simulink model "Twin_Rotor_Mimo_System_Pitch and Yaw Control"  (R2022b)
settings: Solver=VariableStepAuto  StartTime=0.0  StopTime=600
libraries: slpidlib x2
settings Model: SimulationMode=accelerator  Creator=Shaan Sapru  LastModifiedBy=Shaan Sapru
settings SolverCC: ZeroCrossAlgorithm=Adaptive
settings DebuggingCC: IgnoredZcDiagnostic=none

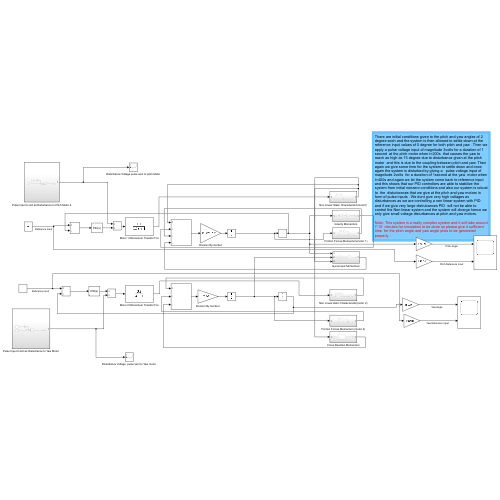
[thumbnail: Simulink's stored preview of the top-level diagram]
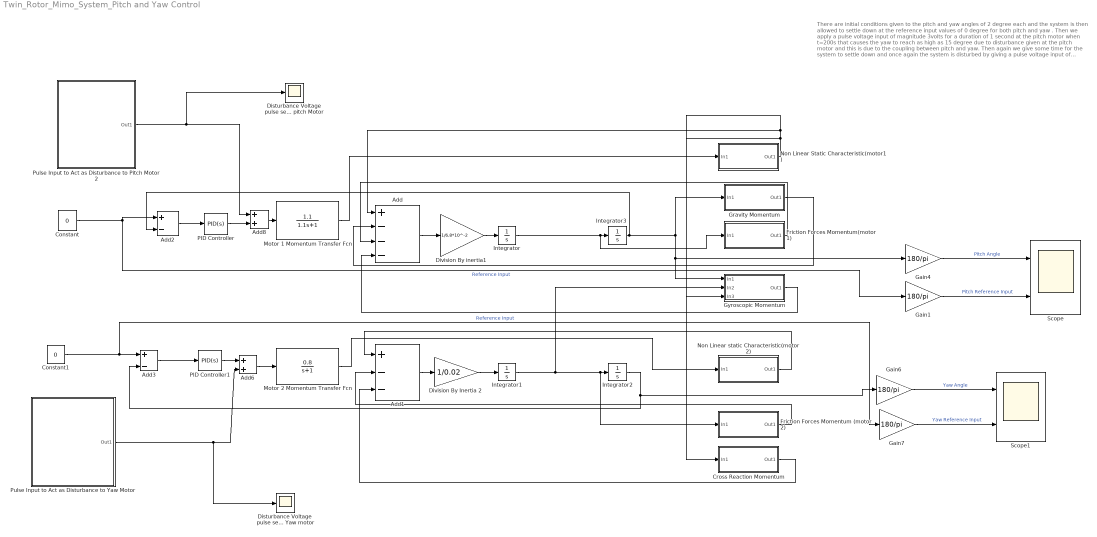
== system Twin_Rotor_Mimo_System_Pitch and Yaw Control ==
  note: There are initial conditions given to the pitch and yaw angles of 2 degree each and the system is then allowed to settle down at the reference input values of 0 degree for both pitch and yaw . Then we apply a pulse voltage input of magnitude 3volts for a duration of 1 second at the pitch motor when t=200s that causes the yaw to reach as high as 15 degree due to disturbance given at the pitch motor and this is due to the coupling between pitch and yaw. Then again we give some time for the system to settle down and once again the system is disturbed by giving a pulse voltage input of magnitude 2volts for a duration of 1second at the yaw motor when t=400s and again we let the system come back to reference input and this shows that our PID controllers are able to stabilize the system from initial nonzero conditions and also our system is robust to the disturbances that we give at the pitch and yaw motors in form of pulse inputs . We dont give very high voltages as disturbances as we are controlling a non linear system with PID and if we give very large distrubances PID will not be able to control the Non linear system and the system will diverge hence we only give small voltage disturbances at pitch and yaw motors.
      |
      | Note- This system is a really complex system and it will take around 7-10 minutes for simulation to be done so please give it sufficient time for the pitch angle and yaw angle plots to be generated properly .
  Add : Sum  Inputs=+---
  Add1 : Sum  Inputs=+--
  Add2 : Sum  Inputs=+-
  Add3 : Sum  Inputs=+-
  Add6 : Sum
  Add8 : Sum
  Constant : Constant  Value=0
  Constant1 : Constant  Value=0
  Cross Reaction Momentum : Subsystem
  "Disturbance Voltage  pulse sent to Yaw motor " : Scope
  Disturbance Voltage pulse sent to pitch Motor : Scope
  Division By Inertia 2 : Gain  Gain=1/0.02
  Division By inertia1 : Gain  Gain=1/6.8*10^-2
  Friction Forces Momentum (motor 2) : Subsystem
  Friction Forces Momentum(motor 1) : Subsystem
  Gain{1,4,6..7} (4 alike) : Gain  Gain=180/pi
  Gravity Momentum : Subsystem
  Gyroscopic Momentum : Subsystem
  Integrator : Integrator
  Integrator1 : Integrator
  Integrator2 : Integrator  InitialCondition=2*(pi/180)
  Integrator3 : Integrator  InitialCondition=2*(pi/180)
  Motor 1 Momentum Transfer Fcn : TransferFcn  Numerator=[1.1]  Denominator="[1.1  1]"
  Motor 2 Momentum Transfer Fcn : TransferFcn  Numerator=[0.8]  Denominator=[1 1]
  Non Linear Static Characteristic(motor1) : Subsystem
  Non Linear static Characteristic(motor 2) : Subsystem
  PID Controller : slpidlib/PID Controller  Controller=PID  Form=Parallel  TimeDomain=Continuous-time  UseExternalTs=off  SampleTime=-1  IntegratorMethod=Forward Euler  FilterMethod=Forward Euler  ControllerParametersSource=internal  P=0.231955535169778  I=5.67987011227532e-05  UseKiTs=off  D=210.470895128174  N=4.7968197094642  UseFilter=on  TunerSelectOption=Transfer Function Based (PID Tuner App)  InitialConditionSource=internal  InitialConditionForIntegrator=0  InitialConditionForFilter=0  DifferentiatorICPrevScaledInput=0  ExternalReset=none  TrackingMode=off  Kt=1  LimitOutput=off  SatLimitsSource=internal  UpperSaturationLimit=inf  LowerSaturationLimit=-inf  LinearizeAsGain=on  AntiWindupMode=none  Kb=1  LimitIntegrator=off  UpperIntegratorSaturationLimit=inf  LowerIntegratorSaturationLimit=-inf  POutMin=[]  POutMax=[]  IOutMin=[]  IOutMax=[]  DOutMin=[]  DOutMax=[]  NOutMin=[]  NOutMax=[]  SumOutMin=[]  SumOutMax=[]  SaturationOutMin=[]  SaturationOutMax=[]  PParamMin=[]  PParamMax=[]  IParamMin=[]  IParamMax=[]  DParamMin=[]  DParamMax=[]  NParamMin=[]  NParamMax=[]  KbParamMin=[]  KbParamMax=[]  KtParamMin=[]  KtParamMax=[]  KbOutMin=[]  KbOutMax=[]  KtOutMin=[]  KtOutMax=[]  IntegratorOutMin=[]  IntegratorOutMax=[]  FilterOutMin=[]  FilterOutMax=[]  SumI1OutMin=[]  SumI1OutMax=[]  SumI2OutMin=[]  SumI2OutMax=[]  SumI3OutMin=[]  SumI3OutMax=[]  SumI4OutMin=[]  SumI4OutMax=[]  SumDOutMin=[]  SumDOutMax=[]  DifferentiatorOutMin=[]  DifferentiatorOutMax=[]  FilterDiffOutCoefMin=[]  FilterDiffOutCoefMax=[]  ReciprocalOutMin=[]  ReciprocalOutMax=[]  SumDenOutMin=[]  SumDenOutMax=[]  SumNumOutMin=[]  SumNumOutMax=[]  DivideOutMin=[]  DivideOutMax=[]  UdiffTsProdOutMin=[]  UdiffTsProdOutMax=[]  NTsProdOutMin=[]  NTsProdOutMax=[]  UintegralTsProdOutMin=[]  UintegralTsProdOutMax=[]  UngainTsProdOutMin=[]  UngainTsProdOutMax=[]  ClampingZeroOutDataTypeStr=Inherit: Inherit via back propagation  ClampingZeroOutMin=[]  ClampingZeroOutMax=[]  FilterDenConstantOutDataTypeStr=Inherit: Inherit via back propagation  FilterDenConstantOutMin=[]  FilterDenConstantOutMax=[]  PCopyOutDataTypeStr=Inherit: Inherit via back propagation  PCopyOutMin=[]  PCopyOutMax=[]  NCopyOutDataTypeStr=Inherit: Inherit via back propagation  NCopyOutMin=[]  NCopyOutMax=[]  IntegratorContinuousStateAttributes=''  IntegratorStateMustResolveToSignalObject=off  IntegratorRTWStateStorageClass=Auto  FilterContinuousStateAttributes=''  FilterStateMustResolveToSignalObject=off  FilterRTWStateStorageClass=Auto  ParallelPVariant=InternalParameters  IdealPVariant=Disabled  IVariant=InternalParameters  DVariant=InternalParameters  IntegratorVariant=Continuous  SatVariant=Disabled  AWVariant=Passthrough  PCopyVariant=Disabled  TRVariant=Disabled  FdbkBlocksVariant=Forward  IdealPFdbkVariant=Disabled  SatFdbkVariant=Disabled  DerivativeFilterVariant=ContFilter  NVariant=InternalParameters  NCopyVariant=Disabled  FilterICVariant=InternalICsFilter  IntegratorICVariant=InternalICs  ExternalResetVariant=Disabled  TRSumVariant=Passthrough  SumFdbkVariant=Disabled  SumVariant=Sum_PID  TsampFilterVariant=InternalTs  TsampNgainVariant=Passthrough  TsampIntegralVariant=Passthrough  ExternalSaturationOutDataTypeStr=Inherit: Same as second input
  PID Controller1 : slpidlib/PID Controller  Controller=PID  Form=Parallel  TimeDomain=Continuous-time  UseExternalTs=off  SampleTime=-1  IntegratorMethod=Forward Euler  FilterMethod=Forward Euler  ControllerParametersSource=internal  P=1.252834869870105  I=0.00741895473472099  UseKiTs=off  D=5.565923160534852  N=1.80905354804325  UseFilter=on  TunerSelectOption=Transfer Function Based (PID Tuner App)  InitialConditionSource=internal  InitialConditionForIntegrator=0  InitialConditionForFilter=0  DifferentiatorICPrevScaledInput=0  ExternalReset=none  TrackingMode=off  Kt=1  LimitOutput=off  SatLimitsSource=internal  UpperSaturationLimit=inf  LowerSaturationLimit=-inf  LinearizeAsGain=on  AntiWindupMode=none  Kb=1  LimitIntegrator=off  UpperIntegratorSaturationLimit=inf  LowerIntegratorSaturationLimit=-inf  POutMin=[]  POutMax=[]  IOutMin=[]  IOutMax=[]  DOutMin=[]  DOutMax=[]  NOutMin=[]  NOutMax=[]  SumOutMin=[]  SumOutMax=[]  SaturationOutMin=[]  SaturationOutMax=[]  PParamMin=[]  PParamMax=[]  IParamMin=[]  IParamMax=[]  DParamMin=[]  DParamMax=[]  NParamMin=[]  NParamMax=[]  KbParamMin=[]  KbParamMax=[]  KtParamMin=[]  KtParamMax=[]  KbOutMin=[]  KbOutMax=[]  KtOutMin=[]  KtOutMax=[]  IntegratorOutMin=[]  IntegratorOutMax=[]  FilterOutMin=[]  FilterOutMax=[]  SumI1OutMin=[]  SumI1OutMax=[]  SumI2OutMin=[]  SumI2OutMax=[]  SumI3OutMin=[]  SumI3OutMax=[]  SumI4OutMin=[]  SumI4OutMax=[]  SumDOutMin=[]  SumDOutMax=[]  DifferentiatorOutMin=[]  DifferentiatorOutMax=[]  FilterDiffOutCoefMin=[]  FilterDiffOutCoefMax=[]  ReciprocalOutMin=[]  ReciprocalOutMax=[]  SumDenOutMin=[]  SumDenOutMax=[]  SumNumOutMin=[]  SumNumOutMax=[]  DivideOutMin=[]  DivideOutMax=[]  UdiffTsProdOutMin=[]  UdiffTsProdOutMax=[]  NTsProdOutMin=[]  NTsProdOutMax=[]  UintegralTsProdOutMin=[]  UintegralTsProdOutMax=[]  UngainTsProdOutMin=[]  UngainTsProdOutMax=[]  ClampingZeroOutDataTypeStr=Inherit: Inherit via back propagation  ClampingZeroOutMin=[]  ClampingZeroOutMax=[]  FilterDenConstantOutDataTypeStr=Inherit: Inherit via back propagation  FilterDenConstantOutMin=[]  FilterDenConstantOutMax=[]  PCopyOutDataTypeStr=Inherit: Inherit via back propagation  PCopyOutMin=[]  PCopyOutMax=[]  NCopyOutDataTypeStr=Inherit: Inherit via back propagation  NCopyOutMin=[]  NCopyOutMax=[]  IntegratorContinuousStateAttributes=''  IntegratorStateMustResolveToSignalObject=off  IntegratorRTWStateStorageClass=Auto  FilterContinuousStateAttributes=''  FilterStateMustResolveToSignalObject=off  FilterRTWStateStorageClass=Auto  ParallelPVariant=InternalParameters  IdealPVariant=Disabled  IVariant=InternalParameters  DVariant=InternalParameters  IntegratorVariant=Continuous  SatVariant=Disabled  AWVariant=Passthrough  PCopyVariant=Disabled  TRVariant=Disabled  FdbkBlocksVariant=Forward  IdealPFdbkVariant=Disabled  SatFdbkVariant=Disabled  DerivativeFilterVariant=ContFilter  NVariant=InternalParameters  NCopyVariant=Disabled  FilterICVariant=InternalICsFilter  IntegratorICVariant=InternalICs  ExternalResetVariant=Disabled  TRSumVariant=Passthrough  SumFdbkVariant=Disabled  SumVariant=Sum_PID  TsampFilterVariant=InternalTs  TsampNgainVariant=Passthrough  TsampIntegralVariant=Passthrough  ExternalSaturationOutDataTypeStr=Inherit: Same as second input
  Pulse Input to Act as Disturbance to Pitch Motor 2 : Subsystem
  Pulse Input to Act as Disturbance to Yaw Motor : Subsystem
  Scope : Scope  NumInputPorts=2
  Scope1 : Scope  NumInputPorts=2
  wires:
  Integrator/1 -> Integrator3/1, Friction Forces Momentum(motor 1)/1(In1)
  Integrator1/1 -> Gyroscopic Momentum/2(In2), Friction Forces Momentum (motor 2)/1(In1), Integrator2/1
  Add1/1 -> Division By Inertia 2/1
  Add/1 -> Division By inertia1/1
  Add3/1 -> PID Controller1/1
  Motor 1 Momentum Transfer Fcn/1 -> Non Linear Static Characteristic(motor1)/1(In1)
  Non Linear Static Characteristic(motor1)/1(Out1) -> Add/1, Cross Reaction Momentum/1(In1), Gyroscopic Momentum/3(In3)
  Integrator3/1 -> Add2/2, Gyroscopic Momentum/1(In1), Gain4/1, Gravity Momentum/1(In1)
  Gravity Momentum/1(Out1) -> Add/2
  Friction Forces Momentum(motor 1)/1(Out1) -> Add/3
  Gyroscopic Momentum/1(Out1) -> Add/4
  Motor 2 Momentum Transfer Fcn/1 -> Non Linear static Characteristic(motor 2)/1(In1)
  Non Linear static Characteristic(motor 2)/1(Out1) -> Add1/1
  Friction Forces Momentum (motor 2)/1(Out1) -> Add1/2
  Cross Reaction Momentum/1(Out1) -> Add1/3
  Integrator2/1 -> Add3/2, Gain6/1
  Constant/1 -> Gain1/1, Add2/1  "Reference Input"
  Division By inertia1/1 -> Integrator/1
  Division By Inertia 2/1 -> Integrator1/1
  Constant1/1 -> Add3/1, Gain7/1  "Reference Input"
  PID Controller1/1 -> Add6/1
  Add6/1 -> Motor 2 Momentum Transfer Fcn/1
  Add2/1 -> PID Controller/1
  PID Controller/1 -> Add8/2
  Add8/1 -> Motor 1 Momentum Transfer Fcn/1
  Gain1/1 -> Scope/2  "Pitch Reference Input"
  Gain4/1 -> Scope/1  "Pitch Angle"
  Gain6/1 -> Scope1/1  "Yaw Angle"
  Gain7/1 -> Scope1/2  "Yaw Reference Input"
  Pulse Input to Act as Disturbance to Yaw Motor/1(Out1) -> Add6/2, "Disturbance Voltage  pulse sent to Yaw motor "/1
  Pulse Input to Act as Disturbance to Pitch Motor 2/1(Out1) -> Add8/1, Disturbance Voltage pulse sent to pitch Motor/1

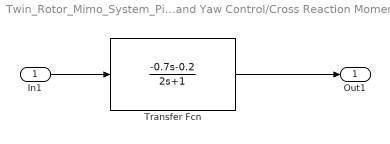
== system Twin_Rotor_Mimo_System_Pitch and Yaw Control/Cross Reaction Momentum ==
  In1 : Inport
  Transfer Fcn : TransferFcn  Numerator=[-0.7 -0.2]  Denominator="[2  1]"
  Out1 : Outport
  wires:
  In1/1 -> Transfer Fcn/1
  Transfer Fcn/1 -> Out1/1

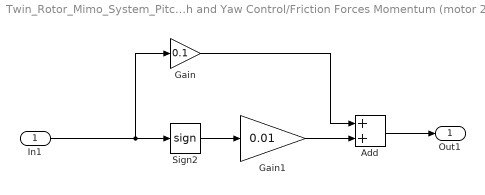
== system Twin_Rotor_Mimo_System_Pitch and Yaw Control/Friction Forces Momentum (motor 2) ==
  In1 : Inport
  Add : Sum
  Gain : Gain  Gain=0.1
  Gain1 : Gain  Gain=0.01
  Sign2 : Signum
  Out1 : Outport
  wires:
  Gain/1 -> Add/1
  Gain1/1 -> Add/2
  Add/1 -> Out1/1
  In1/1 -> Sign2/1, Gain/1
  Sign2/1 -> Gain1/1

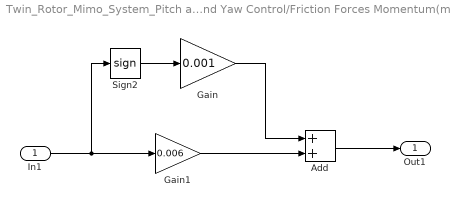
== system Twin_Rotor_Mimo_System_Pitch and Yaw Control/Friction Forces Momentum(motor 1) ==
  In1 : Inport
  Add : Sum
  Gain : Gain  Gain=0.001
  Gain1 : Gain  Gain=0.006
  Sign2 : Signum
  Out1 : Outport
  wires:
  Add/1 -> Out1/1
  Gain1/1 -> Add/2
  Gain/1 -> Add/1
  In1/1 -> Sign2/1, Gain1/1
  Sign2/1 -> Gain/1

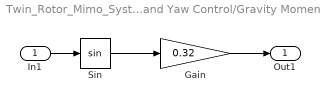
== system Twin_Rotor_Mimo_System_Pitch and Yaw Control/Gravity Momentum ==
  In1 : Inport
  Gain : Gain  Gain=0.32
  Sin : Trigonometry
  Out1 : Outport
  wires:
  In1/1 -> Sin/1
  Gain/1 -> Out1/1
  Sin/1 -> Gain/1

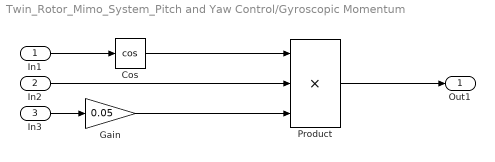
== system Twin_Rotor_Mimo_System_Pitch and Yaw Control/Gyroscopic Momentum ==
  In1 : Inport
  In2 : Inport  Port=2
  In3 : Inport  Port=3
  Cos : Trigonometry  Operator=cos
  Gain : Gain  Gain=0.05
  Product : Product  Inputs=3
  Out1 : Outport
  wires:
  In3/1 -> Gain/1
  Product/1 -> Out1/1
  Gain/1 -> Product/3
  In1/1 -> Cos/1
  Cos/1 -> Product/1
  In2/1 -> Product/2

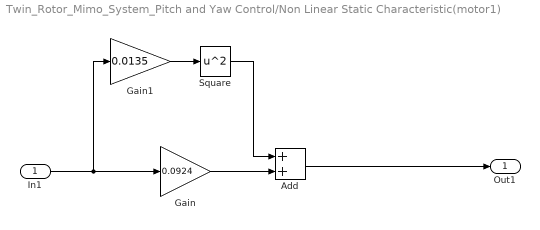
== system Twin_Rotor_Mimo_System_Pitch and Yaw Control/Non Linear Static Characteristic(motor1) ==
  In1 : Inport
  Add : Sum
  Gain : Gain  Gain=0.0924
  Gain1 : Gain  Gain=0.0135
  Square : Math  Operator=square
  Out1 : Outport
  wires:
  In1/1 -> Gain1/1, Gain/1
  Gain1/1 -> Square/1
  Gain/1 -> Add/2
  Square/1 -> Add/1
  Add/1 -> Out1/1

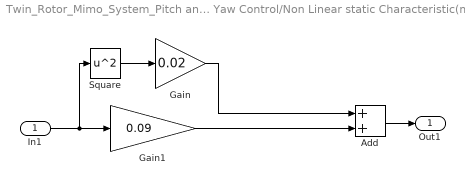
== system Twin_Rotor_Mimo_System_Pitch and Yaw Control/Non Linear static Characteristic(motor 2) ==
  In1 : Inport
  Add : Sum
  Gain : Gain  Gain=0.02
  Gain1 : Gain  Gain=0.09
  Square : Math  Operator=square
  Out1 : Outport
  wires:
  Add/1 -> Out1/1
  In1/1 -> Square/1, Gain1/1
  Gain1/1 -> Add/2
  Square/1 -> Gain/1
  Gain/1 -> Add/1

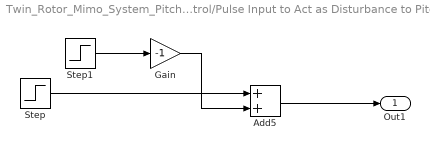
== system Twin_Rotor_Mimo_System_Pitch and Yaw Control/Pulse Input to Act as Disturbance to Pitch Motor 2 ==
  Add5 : Sum
  Gain : Gain  Gain=-1
  Step : Step  Time=200  After=3  SampleTime=0
  Step1 : Step  Time=201  After=3  SampleTime=0
  Out1 : Outport
  wires:
  Step/1 -> Add5/1
  Add5/1 -> Out1/1
  Step1/1 -> Gain/1
  Gain/1 -> Add5/2

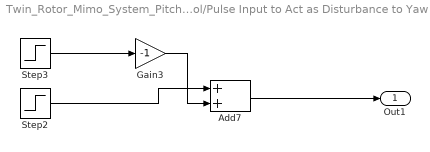
== system Twin_Rotor_Mimo_System_Pitch and Yaw Control/Pulse Input to Act as Disturbance to Yaw Motor ==
  Add7 : Sum
  Gain3 : Gain  Gain=-1
  Step2 : Step  Time=400  After=2  SampleTime=0
  Step3 : Step  Time=401  After=2  SampleTime=0
  Out1 : Outport
  wires:
  Step3/1 -> Gain3/1
  Step2/1 -> Add7/1
  Gain3/1 -> Add7/2
  Add7/1 -> Out1/1
